simulink model "mcb_microchip_pmsm_autotuner_host_SAME70"  (R2023a)
settings: Solver=FixedStepDiscrete  StartTime=0.0  StopTime=inf  RelTol=1e-3  EnableMultiTasking=on
values from neighbouring files (symbols this model uses):
  Ts = T_pwm    (= 5e-05)    [mcb_microchip_pmsm_autotuner_SAME70_data.m]
  Ts_SerialCom = 0.0005    [mcb_microchip_pmsm_autotuner_SAME70_data.m]
undefined symbols (not defined in the file or in its folder): target
libraries: instrumentseriallib x3, simulink x2
settings Model: Creator=The MathWorks, Inc.  LastModifiedBy=snarayan
settings SolverCC: AlgebraicLoopSolver=TrustRegion
settings DataIOCC: LimitDataPoints=on  SaveFormat=Array  ReturnWorkspaceOutputs=off
settings OptimizationCC: LifeSpan=1  EfficientTunableParamExpr=on
settings DebuggingCC: MergeDetectMultiDrivingBlocksExec=none  SolverPrmCheckMsg=warning  ParameterPrecisionLossMsg=none  UnconnectedInputMsg=warning  UnconnectedOutputMsg=warning  UnconnectedLineMsg=warning  AllowSymbolicDim=off  PregeneratedLibrarySubsystemCodeDiagnostic=none  SFUnexpectedBacktrackingDiag=warning  SFNoUnconditionalDefaultTransitionDiag=warning  SFExecutionAtInitializationDiag=none  ArithmeticOperatorsInVariantConditions=warning
settings HardwareCC: ProdBitPerPointer=32  ProdLargestAtomicFloat=None  ProdIntDivRoundTo=Undefined  ProdEndianess=Unspecified  ProdWordSize=32  ProdHWDeviceType=32-bit Generic
settings ModelReferenceCC: EnableRefExpFcnMdlSchedulingChecks=on  PropagateSignalLabelsOutOfModel=off
settings SFSimCC: SimUseLocalCustomCode=off  MATLABDynamicMemAlloc=off
settings RTWCC: Description=Real-Time Workshop Embedded Coder  SystemTargetFile=ert.tlc  TemplateMakefile=ert_default_tmf  GenerateReport=on  RTWUseLocalCustomCode=off  IncludeHyperlinkInReport=on  LaunchReport=on  GenerateTraceInfo=on  GenerateTraceReport=on  GenerateTraceReportSl=on  GenerateTraceReportSf=on  GenerateTraceReportEml=on  DLArmComputeVersion=19.05
settings CodeAppCC: IgnoreCustomStorageClasses=off  StateflowObjectComments=on  InternalIdentifier=Classic
settings ERTTargetCC: MultiwordLength=2048  GenerateSampleERTMain=on  ERTCustomFileTemplate=example_file_process.tlc  ConvertIfToSwitch=off  SuppressUnreachableDefaultCases=off
settings ConfigComp: CovMetricSettings=dw  CovSaveCumulativeToWorkspaceVar=on  CovSaveSingleToWorkspaceVar=on  CovExternalEMLEnable=off  CovSFcnEnable=off

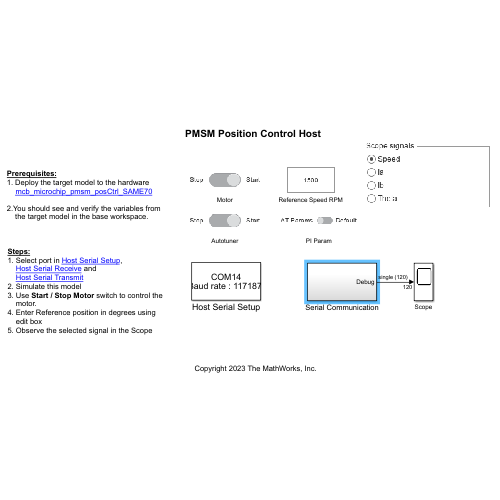
[thumbnail: Simulink's stored preview of the top-level diagram]
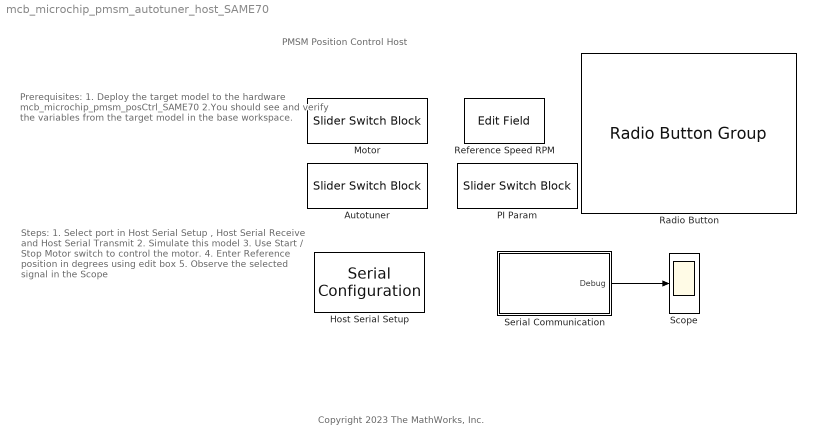
== system mcb_microchip_pmsm_autotuner_host_SAME70 ==
  note: PMSM Position Control Host
  note: Copyright 2023 The MathWorks, Inc.
  note: Prerequisites:
      | 1. Deploy the target model to the hardware
      | mcb_microchip_pmsm_posCtrl_SAME70
      |
      | 2.You should see and verify the variables from
      | the target model in the base workspace.
  note: Steps:
      | 1. Select port in Host Serial Setup ,
      | Host Serial Receive and
      | Host Serial Transmit
      | 2. Simulate this model
      | 3. Use Start / Stop Motor switch to control the
      | motor.
      | 4. Enter Reference position in degrees using
      | edit box
      | 5. Observe the selected signal in the Scope
  Autotuner : SliderSwitchBlock  LabelPosition=Hide
      settings: Values={{'Stop', 'Start'}, [0 1]}
  Host Serial Setup : instrumentseriallib/Serial Configuration  Priority=-99  PortSel=COM14  Port=COM14  ComPort=COM14  BaudRate=1171875  DataBits=8  Parity=none  StopBits=1  ByteOrder=little-endian  FlowControl=none  Timeout=2  SimulateUsing=Interpreted execution  BlockInModel=on  aMode=5
  Motor : SliderSwitchBlock  LabelPosition=Hide
      settings: Values={{'Stop', 'Start'}, [0 1]}
  PI Param : SliderSwitchBlock  LabelPosition=Hide
      settings: Values={{'AT Params', 'Default'}, [0 1]}
  Radio Button : RadioButtonGroup  LabelPosition=Hide  SelectedLabel=Speed  ButtonGroupName=Scope signals
      settings: Values={{'Speed', 'Ia', 'Ib', 'Theta'}, [1 2 3 4]}
  Reference Speed RPM : EditField  LabelPosition=Hide  ShowInitialText=on  Alignment=Center
  Scope : Scope
  Serial Communication : Subsystem
  wires:
  Serial Communication/1(Debug) -> Scope/1

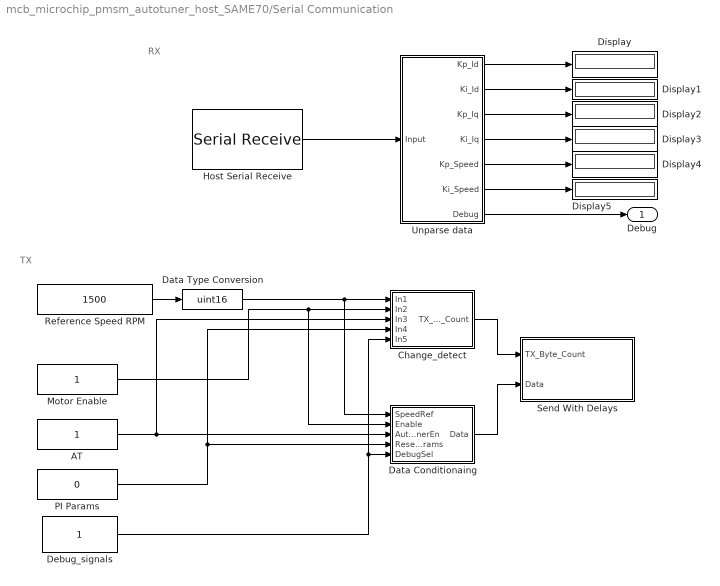
== system mcb_microchip_pmsm_autotuner_host_SAME70/Serial Communication ==
  note: RX
  note: TX
  AT : Constant  VectorParams1D=off  OutDataTypeStr=uint8  SampleTime=600 * Ts
  Change_detect : Subsystem
  Data Conditionaing : Subsystem  VariantControl=~isequal(dataType, 'single')
  Data Type Conversion : DataTypeConversion  OutDataTypeStr=uint16  ConvertRealWorld=Stored Integer (SI)  RndMeth=Simplest  SaturateOnIntegerOverflow=off
  Debug_signals : Constant  OutDataTypeStr=uint8  SampleTime=600 * Ts
  Display{,1..5} (6 alike) : Display
      settings: Decimation=4
  Host Serial Receive : instrumentseriallib/Serial Receive  PortSel=COM14  Port=COM14  ComPort=COM14  DataType=single  SaveDataType=uint8  ToggleHeader=on  Header='ES'  ToggleTerminator=off  Terminator=<none>  CustomTerminator='E'  InputFormat=Row major  ToggleDataSize=on  DataSize=[target.SerialFrameSize 3]  EnableBlockingMode=on  ActionDataUnavailable=Output custom value  ActionWhenDataUnavailable=Output custom value  CustomValue=15  SampleTime=Ts_SerialCom * target.SerialFrameSize  SimulateUsing=Interpreted execution  BlockInModel=on  aMode=5
  Motor Enable : Constant  VectorParams1D=off  OutDataTypeStr=uint8  SampleTime=600 * Ts
  PI Params : Constant  Value=0  VectorParams1D=off  OutDataTypeStr=uint8  SampleTime=600 * Ts
  Reference Speed RPM : Constant  Value=1500  VectorParams1D=off  OutDataTypeStr=int16  SampleTime=600 * Ts
  Send With Delays : Subsystem
  Unparse data : Subsystem
  Debug : Outport
  wires:
  Motor Enable/1 -> Data Conditionaing/2(Enable), Change_detect/2(In2)
  Change_detect/1(TX_Byte_Count) -> Send With Delays/1(TX_Byte_Count)
  Data Conditionaing/1(Data) -> Send With Delays/2(Data)
  Reference Speed RPM/1 -> Data Type Conversion/1
  AT/1 -> Change_detect/3(In3), Data Conditionaing/3(AutoTunerEn)
  PI Params/1 -> Data Conditionaing/4(ResetPIParams), Change_detect/4(In4)
  Debug_signals/1 -> Data Conditionaing/5(DebugSel), Change_detect/5(In5)
  Data Type Conversion/1 -> Data Conditionaing/1(SpeedRef), Change_detect/1(In1)
  Host Serial Receive/1 -> Unparse data/1(Input)
  Unparse data/1(Kp_Id) -> Display/1
  Unparse data/2(Ki_Id) -> Display1/1
  Unparse data/3(Kp_Iq) -> Display2/1
  Unparse data/4(Ki_Iq) -> Display3/1
  Unparse data/5(Kp_Speed) -> Display4/1
  Unparse data/6(Ki_Speed) -> Display5/1
  Unparse data/7(Debug) -> Debug/1

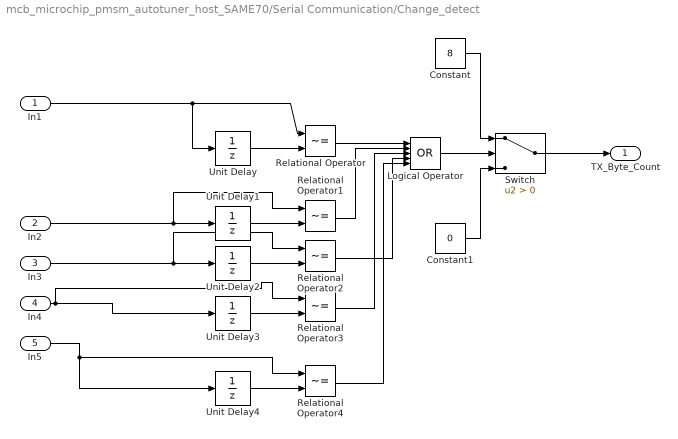
== system mcb_microchip_pmsm_autotuner_host_SAME70/Serial Communication/Change_detect ==
  In1 : Inport
  In2 : Inport  Port=2
  In3 : Inport  Port=3
  In4 : Inport  Port=4
  In5 : Inport  Port=5
  Constant : Constant  Value=8  OutDataTypeStr=uint8
  Constant1 : Constant  Value=0  OutDataTypeStr=uint8
  Logical Operator : Logic  Operator=OR  Inputs=5  AllPortsSameDT=off  OutDataTypeStr=boolean
  Relational Operator{,1..4} (5 alike) : RelationalOperator  Operator=~=  OutDataTypeStr=boolean  InputSameDT=off
  Switch : Switch  Criteria=u2 > Threshold  SaturateOnIntegerOverflow=off  InputSameDT=off
  Unit Delay : UnitDelay  InitialCondition=0.5  SampleTime=-1  HasFrameUpgradeWarning=on
  Unit Delay{1..4} (4 alike) : UnitDelay  SampleTime=-1  HasFrameUpgradeWarning=on
  TX_Byte_Count : Outport  VectorParamsAs1DForOutWhenUnconnected=off
  wires:
  Relational Operator/1 -> Logical Operator/1
  In1/1 -> Relational Operator/1, Unit Delay/1
  Unit Delay/1 -> Relational Operator/2
  Unit Delay1/1 -> Relational Operator1/2
  Relational Operator1/1 -> Logical Operator/2
  In2/1 -> Unit Delay1/1, Relational Operator1/1
  Constant1/1 -> Switch/3
  Constant/1 -> Switch/1
  Logical Operator/1 -> Switch/2
  Switch/1 -> TX_Byte_Count/1
  In3/1 -> Relational Operator2/1, Unit Delay2/1
  Relational Operator2/1 -> Logical Operator/4
  Unit Delay2/1 -> Relational Operator2/2
  Unit Delay3/1 -> Relational Operator3/2
  Relational Operator3/1 -> Logical Operator/3
  In4/1 -> Relational Operator3/1, Unit Delay3/1
  In5/1 -> Unit Delay4/1, Relational Operator4/1
  Relational Operator4/1 -> Logical Operator/5
  Unit Delay4/1 -> Relational Operator4/2

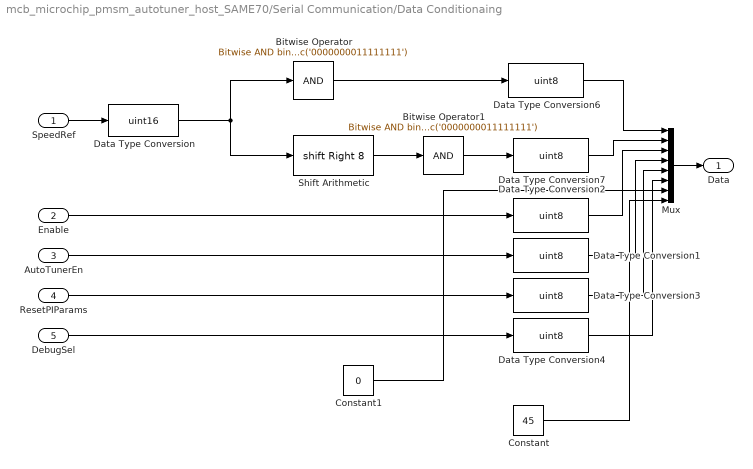
== system mcb_microchip_pmsm_autotuner_host_SAME70/Serial Communication/Data Conditionaing ==
  SpeedRef : Inport
  Enable : Inport  Port=2
  AutoTunerEn : Inport  Port=3
  ResetPIParams : Inport  Port=4
  DebugSel : Inport  Port=5
  Bitwise Operator : simulink/Logic and Bit Operations/Bitwise Operator  logicop=AND  UseBitMask=on  BitMask=bin2dec('0000000011111111')  BitMaskRealWorld=Stored Integer
  Bitwise Operator1 : simulink/Logic and Bit Operations/Bitwise Operator  logicop=AND  UseBitMask=on  BitMask=bin2dec('0000000011111111')  BitMaskRealWorld=Stored Integer
  Constant : Constant  Value=45  OutDataTypeStr=uint8
  Constant1 : Constant  Value=0  OutDataTypeStr=uint8
  Data Type Conversion : DataTypeConversion  OutDataTypeStr=uint16  ConvertRealWorld=Stored Integer (SI)  RndMeth=Simplest  SaturateOnIntegerOverflow=off
  Data Type Conversion{1..4,6..7} (6 alike) : DataTypeConversion  OutDataTypeStr=uint8  RndMeth=Simplest  SaturateOnIntegerOverflow=off
  Mux : Mux  Inputs=8
  Shift Arithmetic : ArithShift  BitShiftNumber=8  BitShiftDirection=Right
  Data : Outport
  wires:
  Mux/1 -> Data/1
  Data Type Conversion6/1 -> Mux/1
  SpeedRef/1 -> Data Type Conversion/1
  Data Type Conversion/1 -> Shift Arithmetic/1, Bitwise Operator/1
  Bitwise Operator/1 -> Data Type Conversion6/1
  Shift Arithmetic/1 -> Bitwise Operator1/1
  Bitwise Operator1/1 -> Data Type Conversion7/1
  Data Type Conversion7/1 -> Mux/2
  Data Type Conversion2/1 -> Mux/3
  Enable/1 -> Data Type Conversion2/1
  AutoTunerEn/1 -> Data Type Conversion1/1
  ResetPIParams/1 -> Data Type Conversion3/1
  DebugSel/1 -> Data Type Conversion4/1
  Constant/1 -> Mux/8
  Constant1/1 -> Mux/7
  Data Type Conversion1/1 -> Mux/4
  Data Type Conversion3/1 -> Mux/5
  Data Type Conversion4/1 -> Mux/6

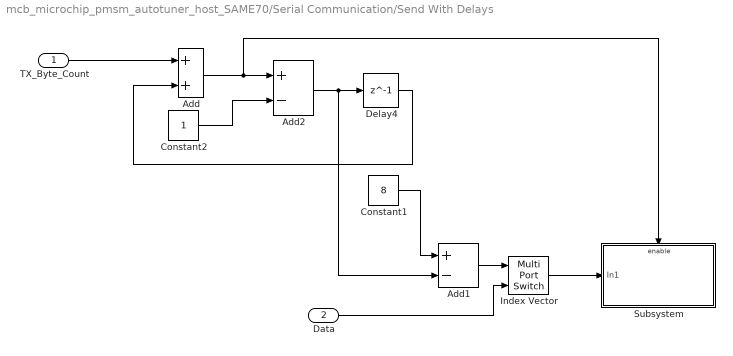
== system mcb_microchip_pmsm_autotuner_host_SAME70/Serial Communication/Send With Delays ==
  TX_Byte_Count : Inport
  Data : Inport  Port=2
  Add : Sum  SaturateOnIntegerOverflow=on
  Add1 : Sum  Inputs=+-  SaturateOnIntegerOverflow=on
  Add2 : Sum  Inputs=+-  SaturateOnIntegerOverflow=on
  Constant1 : Constant  Value=8  OutDataTypeStr=uint8
  Constant2 : Constant  OutDataTypeStr=uint8
  Delay4 : Delay  DelayLength=1
  Index Vector : MultiPortSwitch  Inputs=1  SaturateOnIntegerOverflow=off  InputSameDT=off
  Subsystem : Subsystem
  wires:
  Data/1 -> Index Vector/2
  TX_Byte_Count/1 -> Add/1
  Add/1 -> Subsystem/Enable, Add2/1
  Delay4/1 -> Add/2
  Add1/1 -> Index Vector/1
  Constant1/1 -> Add1/1
  Index Vector/1 -> Subsystem/1(In1)
  Add2/1 -> Add1/2, Delay4/1
  Constant2/1 -> Add2/2

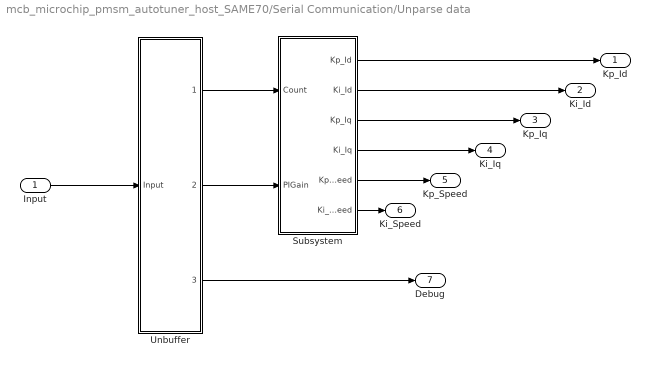
== system mcb_microchip_pmsm_autotuner_host_SAME70/Serial Communication/Unparse data ==
  Input : Inport
  Subsystem : Subsystem
  Unbuffer : MATLAB Function  TreatAsAtomicUnit=on
  Kp_Id : Outport
  Ki_Id : Outport  Port=2
  Kp_Iq : Outport  Port=3
  Ki_Iq : Outport  Port=4
  Kp_Speed : Outport  Port=5
  Ki_Speed : Outport  Port=6
  Debug : Outport  Port=7
  wires:
  Unbuffer/1(Output1) -> Subsystem/1(Count)
  Subsystem/3(Kp_Iq) -> Kp_Iq/1
  Subsystem/5(Kp_Speed) -> Kp_Speed/1
  Subsystem/6(Ki_Speed) -> Ki_Speed/1
  Subsystem/2(Ki_Id) -> Ki_Id/1
  Subsystem/1(Kp_Id) -> Kp_Id/1
  Subsystem/4(Ki_Iq) -> Ki_Iq/1
  Input/1 -> Unbuffer/1(Input)
  Unbuffer/2(Output2) -> Subsystem/2(PIGain)
  Unbuffer/3(Output3) -> Debug/1

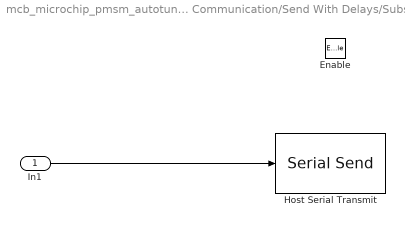
== system mcb_microchip_pmsm_autotuner_host_SAME70/Serial Communication/Send With Delays/Subsystem ==
  In1 : Inport
  Enable : EnablePort
  Host Serial Transmit : instrumentseriallib/Serial Send  PortSel=COM14  Port=COM14  ComPort=COM14  Header=[]  Terminator=<none>  CustomTerminator=[]  EnableBlockingMode=off  SimulateUsing=Interpreted execution  BlockInModel=on  aMode=5
  wires:
  In1/1 -> Host Serial Transmit/1

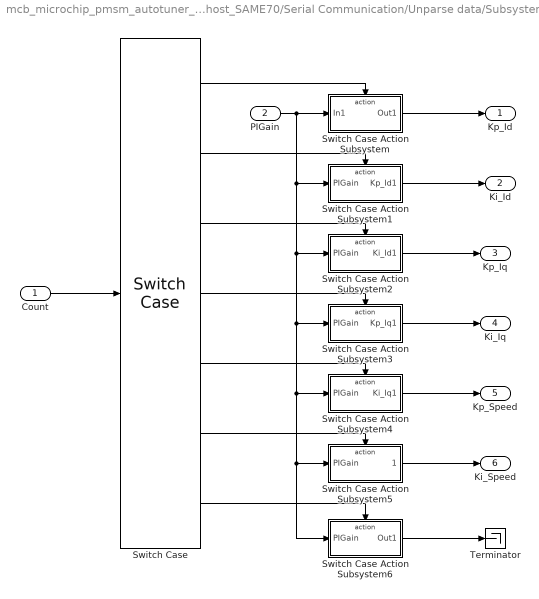
== system mcb_microchip_pmsm_autotuner_host_SAME70/Serial Communication/Unparse data/Subsystem ==
  Count : Inport
  PIGain : Inport  Port=2
  Switch Case : SwitchCase  CaseConditions={1, 2, 3, 4, 5, 6}
  Switch Case Action Subsystem : Subsystem  TreatAsAtomicUnit=on
  Switch Case Action Subsystem1 : Subsystem  TreatAsAtomicUnit=on
  Switch Case Action Subsystem2 : Subsystem  TreatAsAtomicUnit=on
  Switch Case Action Subsystem3 : Subsystem  TreatAsAtomicUnit=on
  Switch Case Action Subsystem4 : Subsystem  TreatAsAtomicUnit=on
  Switch Case Action Subsystem5 : Subsystem  TreatAsAtomicUnit=on
  Switch Case Action Subsystem6 : Subsystem  TreatAsAtomicUnit=on
  Terminator : Terminator
  Kp_Id : Outport
  Ki_Id : Outport  Port=2
  Kp_Iq : Outport  Port=3
  Ki_Iq : Outport  Port=4
  Kp_Speed : Outport  Port=5
  Ki_Speed : Outport  Port=6
  wires:
  Count/1 -> Switch Case/1
  Switch Case/1 -> Switch Case Action Subsystem/Action
  PIGain/1 -> Switch Case Action Subsystem6/1(PIGain), Switch Case Action Subsystem5/1(PIGain), Switch Case Action Subsystem4/1(PIGain), Switch Case Action Subsystem3/1(PIGain), Switch Case Action Subsystem2/1(PIGain), Switch Case Action Subsystem1/1(PIGain), Switch Case Action Subsystem/1(In1)
  Switch Case/2 -> Switch Case Action Subsystem1/Action
  Switch Case/3 -> Switch Case Action Subsystem2/Action
  Switch Case/4 -> Switch Case Action Subsystem3/Action
  Switch Case/5 -> Switch Case Action Subsystem4/Action
  Switch Case/6 -> Switch Case Action Subsystem5/Action
  Switch Case/7 -> Switch Case Action Subsystem6/Action
  Switch Case Action Subsystem/1(Out1) -> Kp_Id/1
  Switch Case Action Subsystem1/1(Kp_Id1) -> Ki_Id/1
  Switch Case Action Subsystem2/1(Ki_Id1) -> Kp_Iq/1
  Switch Case Action Subsystem3/1(Kp_Iq1) -> Ki_Iq/1
  Switch Case Action Subsystem4/1(Ki_Iq1) -> Kp_Speed/1
  Switch Case Action Subsystem5/1(Kp_Speed1) -> Ki_Speed/1
  Switch Case Action Subsystem6/1(Out1) -> Terminator/1

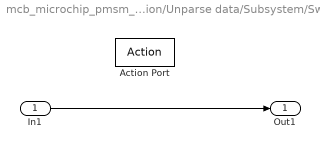
== system mcb_microchip_pmsm_autotuner_host_SAME70/Serial Communication/Unparse data/Subsystem/Switch Case Action Subsystem ==
  In1 : Inport
  Action Port : ActionPort  ActionPortLabel=case [ 1 ]:
  Out1 : Outport
  wires:
  In1/1 -> Out1/1

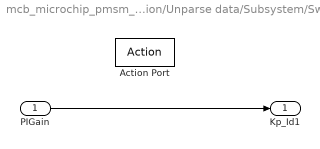
== system mcb_microchip_pmsm_autotuner_host_SAME70/Serial Communication/Unparse data/Subsystem/Switch Case Action Subsystem1 ==
  PIGain : Inport
  Action Port : ActionPort  ActionPortLabel=case [ 2 ]:
  Kp_Id1 : Outport
  wires:
  PIGain/1 -> Kp_Id1/1

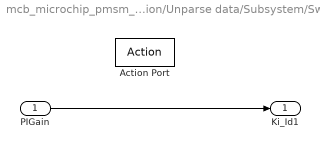
== system mcb_microchip_pmsm_autotuner_host_SAME70/Serial Communication/Unparse data/Subsystem/Switch Case Action Subsystem2 ==
  PIGain : Inport
  Action Port : ActionPort  ActionPortLabel=case [ 3 ]:
  Ki_Id1 : Outport
  wires:
  PIGain/1 -> Ki_Id1/1

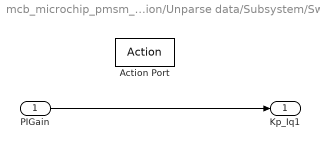
== system mcb_microchip_pmsm_autotuner_host_SAME70/Serial Communication/Unparse data/Subsystem/Switch Case Action Subsystem3 ==
  PIGain : Inport
  Action Port : ActionPort  ActionPortLabel=case [ 4 ]:
  Kp_Iq1 : Outport
  wires:
  PIGain/1 -> Kp_Iq1/1

== system mcb_microchip_pmsm_autotuner_host_SAME70/Serial Communication/Unparse data/Subsystem/Switch Case Action Subsystem4 ==
  PIGain : Inport
  Action Port : ActionPort  ActionPortLabel=case [ 5 ]:
  Ki_Iq1 : Outport
  wires:
  PIGain/1 -> Ki_Iq1/1

== system mcb_microchip_pmsm_autotuner_host_SAME70/Serial Communication/Unparse data/Subsystem/Switch Case Action Subsystem5 ==
  PIGain : Inport
  Action Port : ActionPort  ActionPortLabel=case [ 6 ]:
  Kp_Speed1 : Outport
  wires:
  PIGain/1 -> Kp_Speed1/1

== system mcb_microchip_pmsm_autotuner_host_SAME70/Serial Communication/Unparse data/Subsystem/Switch Case Action Subsystem6 ==
  PIGain : Inport
  Action Port : ActionPort  ActionPortLabel=default:
  Out1 : Outport
  wires:
  PIGain/1 -> Out1/1

== matlab function mcb_microchip_pmsm_autotuner_host_SAME70/Serial Communication/Unparse data/Unbuffer ==
  data: Input input; Output1 output; Output2 output; Output3 output
function [ Output1, Output2, Output3] = unBuf(Input)

selSignal = Input(:, 1);
Output1= selSignal(1,1);

selSignal = Input(:, 2);
Output2 = selSignal(1,1);

Output3 = Input(:, 3);

end
